simulink model "part2_PID_feedback_control"  (R2020b)
settings: Solver=FixedStepAuto  StartTime=0.0  StopTime=1500  FixedStep=0.01  RelTol=1e-3
values from neighbouring files (symbols this model uses):
  ceta = 3    [part1_test_K1.m]    (also in part2_PID_feedback.m)
  cp = 1    [part2_PID_feedback.m]
  K1 = i + (300-length_iter/2)    [part1_test_K1.m]    (also in part2_PID_feedback.m = 0.1)
  K2 = 0.05    [part1_test_K1.m]    (also in part2_PID_feedback.m)
  T = 20    [part1_test_K1.m]    (also in part2_PID_feedback.m)
  tao = 5    [part1_test_K1.m]    (also in part2_PID_feedback.m)
  Thot_air = 35    [part2_PID_feedback.m]
libraries: pid_lib x1
settings Model: Creator=Weiyang  LastModifiedBy=jiang
settings DataIOCC: ReturnWorkspaceOutputs=off

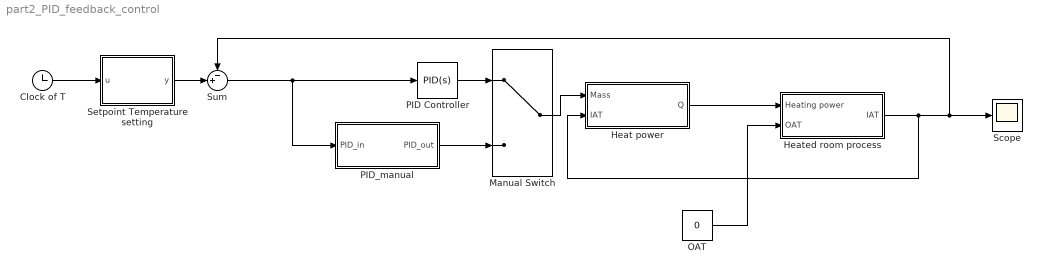
== system part2_PID_feedback_control ==
  Clock of T : Clock
      settings: Decimation=1500
  Heat power : Subsystem
  Heated room process : Subsystem
  Manual Switch : ManualSwitch
  OAT : Constant  Value=0
  PID Controller : pid_lib/PID Controller  Controller=PID  Form=Parallel  TimeDomain=Continuous-time  UseExternalTs=off  SampleTime=-1  IntegratorMethod=Forward Euler  FilterMethod=Forward Euler  ControllerParametersSource=internal  P=1.29516734277125  I=0.0379756826751699  D=8.902214975738  UseFilter=on  N=0.438186898444381  TunerSelectOption=Transfer Function Based (PID Tuner App)  InitialConditionSource=internal  InitialConditionForIntegrator=0  InitialConditionForFilter=0  DifferentiatorICPrevScaledInput=0  ExternalReset=none  TrackingMode=off  Kt=1  LimitOutput=off  SatLimitsSource=internal  UpperSaturationLimit=inf  LowerSaturationLimit=-inf  LinearizeAsGain=on  AntiWindupMode=none  Kb=1  POutMin=[]  POutMax=[]  IOutMin=[]  IOutMax=[]  DOutMin=[]  DOutMax=[]  NOutMin=[]  NOutMax=[]  SumOutMin=[]  SumOutMax=[]  SaturationOutMin=[]  SaturationOutMax=[]  PParamMin=[]  PParamMax=[]  IParamMin=[]  IParamMax=[]  DParamMin=[]  DParamMax=[]  NParamMin=[]  NParamMax=[]  KbParamMin=[]  KbParamMax=[]  KtParamMin=[]  KtParamMax=[]  KbOutMin=[]  KbOutMax=[]  KtOutMin=[]  KtOutMax=[]  IntegratorOutMin=[]  IntegratorOutMax=[]  FilterOutMin=[]  FilterOutMax=[]  SumI1OutMin=[]  SumI1OutMax=[]  SumI2OutMin=[]  SumI2OutMax=[]  SumI3OutMin=[]  SumI3OutMax=[]  SumI4OutMin=[]  SumI4OutMax=[]  SumDOutMin=[]  SumDOutMax=[]  DifferentiatorOutMin=[]  DifferentiatorOutMax=[]  FilterDiffOutCoefMin=[]  FilterDiffOutCoefMax=[]  ReciprocalOutMin=[]  ReciprocalOutMax=[]  SumDenOutMin=[]  SumDenOutMax=[]  SumNumOutMin=[]  SumNumOutMax=[]  DivideOutMin=[]  DivideOutMax=[]  UdiffTsProdOutMin=[]  UdiffTsProdOutMax=[]  NTsProdOutMin=[]  NTsProdOutMax=[]  UintegralTsProdOutMin=[]  UintegralTsProdOutMax=[]  UngainTsProdOutMin=[]  UngainTsProdOutMax=[]  IntegratorContinuousStateAttributes=''  IntegratorStateMustResolveToSignalObject=off  IntegratorRTWStateStorageClass=Auto  FilterContinuousStateAttributes=''  FilterStateMustResolveToSignalObject=off  FilterRTWStateStorageClass=Auto  ParallelPVariant=InternalParameters  IdealPVariant=Disabled  IVariant=InternalParameters  DVariant=InternalParameters  IntegratorVariant=Continuous  SatVariant=Disabled  AWVariant=Passthrough  PCopyVariant=Disabled  TRVariant=Disabled  FdbkBlocksVariant=Forward  IdealPFdbkVariant=Disabled  SatFdbkVariant=Disabled  DerivativeFilterVariant=ContFilter  NVariant=InternalParameters  NCopyVariant=Disabled  FilterICVariant=InternalICsFilter  IntegratorICVariant=InternalICs  ExternalResetVariant=Disabled  TRSumVariant=Passthrough  SumFdbkVariant=Disabled  SumVariant=Sum_PID  TsampFilterVariant=InternalTs  TsampNgainVariant=Passthrough  TsampIntegralVariant=Passthrough  ExternalSaturationOutDataTypeStr=Inherit: Same as second input
  PID_manual : Subsystem
  Scope : Scope
  Setpoint Temperature setting : MATLAB Function  TreatAsAtomicUnit=on
  Sum : Sum  Inputs=-+|
  wires:
  OAT/1 -> Heated room process/2(OAT)
  Sum/1 -> PID Controller/1, PID_manual/1(PID_in)
  Heated room process/1(IAT) -> Heat power/2(IAT), Scope/1, Sum/1
  Clock of T/1 -> Setpoint Temperature setting/1(u)
  Setpoint Temperature setting/1(y) -> Sum/2
  PID Controller/1 -> Manual Switch/1
  Manual Switch/1 -> Heat power/1(Mass)
  Heat power/1(Q) -> Heated room process/1(Heating power)
  PID_manual/1(PID_out) -> Manual Switch/2

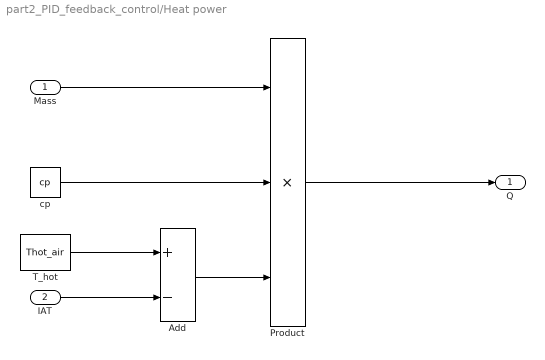
== system part2_PID_feedback_control/Heat power ==
  Mass : Inport
  IAT : Inport  Port=2
  Add : Sum  Inputs=+-
  Product : Product  Inputs=3
  T_hot : Constant  Value=Thot_air
  cp : Constant  Value=cp
  Q : Outport
  wires:
  T_hot/1 -> Add/1
  IAT/1 -> Add/2
  Mass/1 -> Product/1
  cp/1 -> Product/2
  Add/1 -> Product/3
  Product/1 -> Q/1

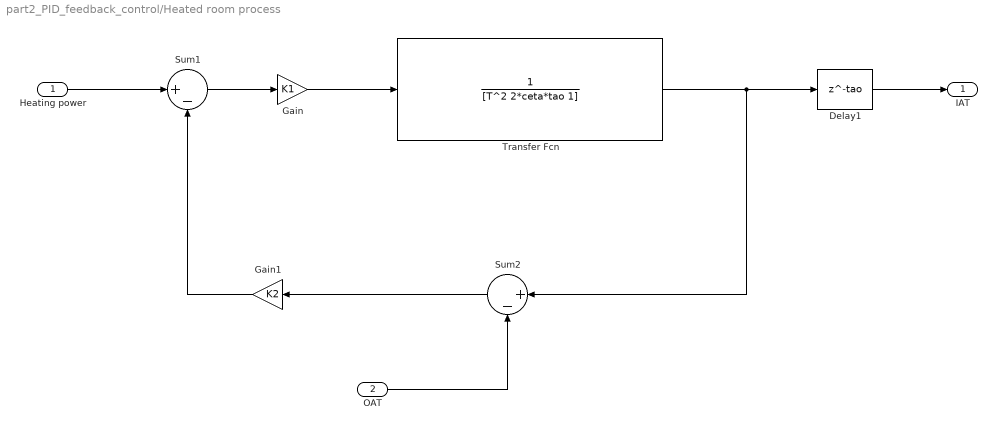
== system part2_PID_feedback_control/Heated room process ==
  Heating power : Inport
  OAT : Inport  Port=2
  Delay1 : Delay  DelayLength=tao  InputProcessing=Columns as channels (frame based)
  Gain : Gain  Gain=K1
  Gain1 : Gain  Gain=K2
  Sum1 : Sum  Inputs=|+-
  Sum2 : Sum  Inputs=|+-
  Transfer Fcn : TransferFcn  Denominator=[T^2 2*ceta*tao 1]
  IAT : Outport
  wires:
  Sum1/1 -> Gain/1
  Gain1/1 -> Sum1/2
  Gain/1 -> Transfer Fcn/1
  Transfer Fcn/1 -> Sum2/1, Delay1/1
  Sum2/1 -> Gain1/1
  Heating power/1 -> Sum1/1
  OAT/1 -> Sum2/2
  Delay1/1 -> IAT/1

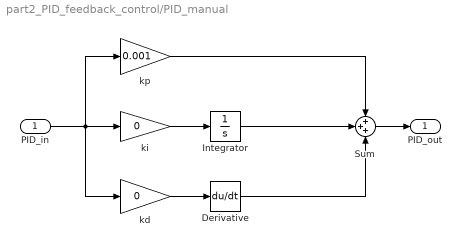
== system part2_PID_feedback_control/PID_manual ==
  PID_in : Inport
  Derivative : Derivative
  Integrator : Integrator
  Sum : Sum  Inputs=+++
  kd : Gain  Gain=0
  ki : Gain  Gain=0
  kp : Gain  Gain=0.001
  PID_out : Outport
  wires:
  PID_in/1 -> kd/1, ki/1, kp/1
  kp/1 -> Sum/1
  Integrator/1 -> Sum/2
  Derivative/1 -> Sum/3
  ki/1 -> Integrator/1
  Sum/1 -> PID_out/1
  kd/1 -> Derivative/1

== matlab function part2_PID_feedback_control/Setpoint Temperature setting ==
  data: u input; y output
function y = fcn(u)
if u>=500&u<1000
    y = 22;
else
    y = 20;
end
end
